simulink model "Simulation_nodeadzone_nodelay"  (R2022b)
settings: Solver=VariableStepAuto  StartTime=0.0  StopTime=24*60*60  RelTol=1e-3
libraries: cstblocks x1
settings Model: Creator=Joy  LastModifiedBy=Hales
settings SolverCC: AlgebraicLoopSolver=TrustRegion
settings DebuggingCC: UnconnectedInputMsg=warning  UnconnectedOutputMsg=warning  UnconnectedLineMsg=warning  SFMachineParentedDataDiag=warning
settings ModelReferenceCC: EnableRefExpFcnMdlSchedulingChecks=on
settings RTWCC: DLArmComputeVersion=19.05

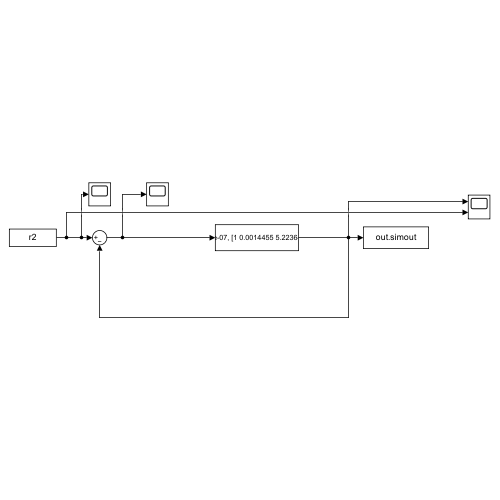
[thumbnail: Simulink's stored preview of the top-level diagram]
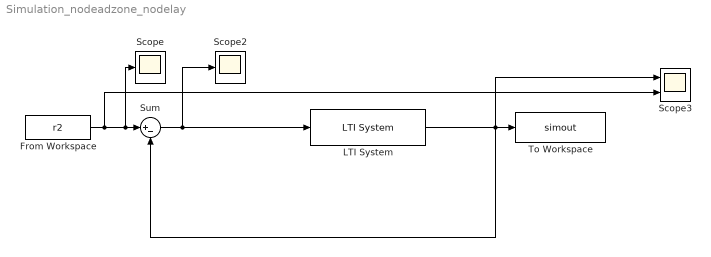
== system Simulation_nodeadzone_nodelay ==
  From Workspace : FromWorkspace  VariableName=r2  SampleTime=60*2.5
  LTI System : cstblocks/LTI System  sys=tf(5.087e-07, [1 0.0014455 5.223645e-07])  IC=[]
  Scope : Scope
  Scope2 : Scope
  Scope3 : Scope  NumInputPorts=2
  Sum : Sum  Inputs=|+-
  To Workspace : ToWorkspace  VariableName=simout  SaveFormat=Timeseries  SampleTime=60*2.5
  wires:
  Sum/1 -> LTI System/1, Scope2/1
  From Workspace/1 -> Scope3/2, Scope/1, Sum/1
  LTI System/1 -> Sum/2, Scope3/1, To Workspace/1
